simulink model "sparam_filter"  (Simulink 6.0)
settings: Solver=ode45  StartTime=0.0  StopTime=10  RelTol=1e-3
undefined symbols (not defined in the file or in its folder): Fs, read, rfdata
libraries: rfports1 x2, rfblackbox1 x1, simulink x1, dspsnks4 x1, dspsrcs4 x1
settings Model: Creator=mikem  LastModifiedBy=rzeng  ProdHWDeviceType=Specified
settings DataIOCC: SaveOutput=off  SaveTime=off  SignalLoggingName=sigsOut
settings DebuggingCC: CheckExecutionContextPreStartOutputMsg=on  CheckExecutionContextRuntimeOutputMsg=on  SolverPrmCheckMsg=none
settings HardwareCC: ProdHWDeviceType=Specified
settings ModelReferenceCC: UpdateModelReferenceTargets=IfOutOfDate
settings SFSimCC: SFSimApplyToAllLibs=on  SFSimBuildMode=Incremental

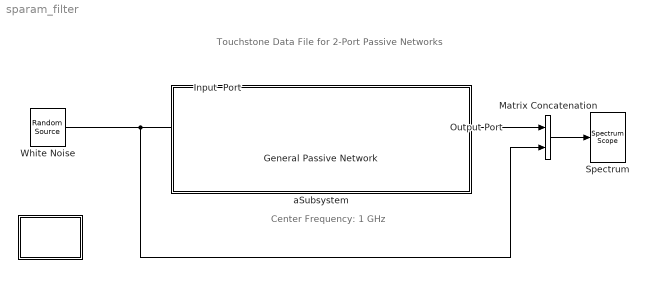
== system sparam_filter ==
  note: Touchstone Data File for 2-Port Passive Networks
  note: Center Frequency: 1 GHz
  " " : Subsystem  PropExecContextAcrossSSBoundary=on
      mask Type: Interpolation filter info block
      mask Display: disp('Info')
  General Passive Network : rfblackbox1/General Passive Network  PhysicalDomain=rfsystemsdomain  SubClassName=general-passive-network  LeftPortType=p1  RightPortType=p1  LConnTagsString=__newl0  RConnTagsString=__newr0  RFDATA=read(rfdata.data, 'passive.s2p')  InterpMethod=Linear  DisplayData=off  PlotFreq=Derived from Input Port parameters  PlotFreqNoSim=Extracted from RFDATA object  Freq=[0.3e6:0.1e6:6e9]  AllPlotType=Composite data  NetworkData=S21  SmithData=S11  PolarData=S11  ComplexFormat=Magnitude (decibels)  DBFormat=Magnitude (decibels)  NoneFormat=None
  Input  Port : rfports1/Input Port  Description=source block  MaxLength=128  Fc=1e9  Ts=0.5e-9  Zs=50  NoiseFlag=off  seed=67987  GoToTag=BABDICLNDBSPFUINKIUJCFB
  Matrix Concatenation : simulink/Math Operations/Matrix Concatenation  numInports=2  catMethod=Horizontal
  Output Port : rfports1/Output Port  Zl=50  num_Models=1  GoToTag=BABDICLNDBSPFUINKIUJCFB  DisplayData=off  PlotFreq=Derived from Input Port parameters  Freq=1e9:1e8:3e9  AllPlotType=Composite data  NoBudgetPlot=Composite data  NetworkData=S11  SmithData=S11  PolarData=S11  ComplexFormat=Magnitude (decibels)  DBFormat=Magnitude (decibels)  DBMFormat=dBm  NoneFormat=None
  Spectrum : dspsnks4/Spectrum Scope  ScopeProperties=on  Domain=Frequency  HorizSpan=1  UseBuffer=on  BufferSize=1024  Overlap=512  inpFftLenInherit=on  FFTlength=1024  numAvg=100  DisplayProperties=off  AxisGrid=on  Memory=off  FrameNumber=on  AxisLegend=off  AxisZoom=off  OpenScopeAtSimStart=on  OpenScopeImmediately=off  FigPos=[6 282 403 292]  AxisProperties=off  XUnits=Hertz  XRange=[-Fs/2...Fs/2]  InheritXIncr=on  XIncr=1.0  XLabel=Samples  YUnits=dB  YLabel=Magnitude, dB  LineProperties=off  LineStyles=--  LineColors=|[1 0 0]
      settings: YMin=-29.8141631310814  YMax=2.51927151651979
  White Noise : dspsrcs4/Random Source  SrcType=Gaussian  NormMethod=Ziggurat  CltLength=12  Min=-1.25  Max=1.25  Mean=0  Var=1  RepMode=Not repeatable  rawSeed=1  Inherit=off  SampMode=Discrete  SampTime=0.5e-9  SampFrame=256  DataType=Double  OutComplex=Complex
  aSubsystem : Subsystem  PropExecContextAcrossSSBoundary=on
      mask Display: disp('')
  wires:
  White Noise/1 -> Input  Port/1, Matrix Concatenation/2
  Matrix Concatenation/1 -> Spectrum/1
  Output Port/1 -> Matrix Concatenation/1
  connections:
  Input  Port/RConn1 -- General Passive Network/LConn1
  General Passive Network/RConn1 -- Output Port/LConn1

== system sparam_filter/  ==
  note: Touchstone Data File for 2-Port Passive Networks
      |
      | The Black Box Elements library has blocks to handle
      | S, Y, and Z parameters of the passive networks.
      | The library also has 'General Passive Network' block
      | that can be used for the Touchstone data file.
      |
      | The data file: 'passive.s2p' has
      | the S-parameters of a 2-port passive network
      | over the frequency range 315KHz to 6GHz.
      | The spectrum plot shows frequency ranging from
      | 0Hz to 2GHz centered at 1GHz.
      |
      |
      | If you want to see the frequency response centered at other RF frequency,
      | you need to change the Center frequency parameter in the
      | 'Input Port' block.
      |
      | If you want to change the range of frequency response that is determined by
      | the Sample time parameter specified in the 'Input Port' and 'White Noise' blocks,
      | you need to change the Sample time parameter in both blocks.

== system sparam_filter/aSubsystem ==
